simulink model "comparison_amp"  (Simulink 6.0)
settings: Solver=ode45  StartTime=0.0  StopTime=10.0  RelTol=1e-3
undefined symbols (not defined in the file or in its folder): dTypeID, Fs, read, rfdata
libraries: rfports1 x6, simulink x3, rfamplifiers1 x3, rfmathmodels1 x2, dspsnks4 x2, dspmtrx3 x1
settings Model: Creator=ashivapr  LastModifiedBy=rzeng  ProdHWDeviceType=Specified
settings DataIOCC: SaveOutput=off  SaveTime=off  SignalLoggingName=logsOut
settings DebuggingCC: CheckExecutionContextPreStartOutputMsg=on  CheckExecutionContextRuntimeOutputMsg=on  SolverPrmCheckMsg=none
settings HardwareCC: ProdHWDeviceType=Specified
settings ModelReferenceCC: UpdateModelReferenceTargets=IfOutOfDate
settings SFSimCC: SFSimApplyToAllLibs=on  SFSimBuildMode=Incremental

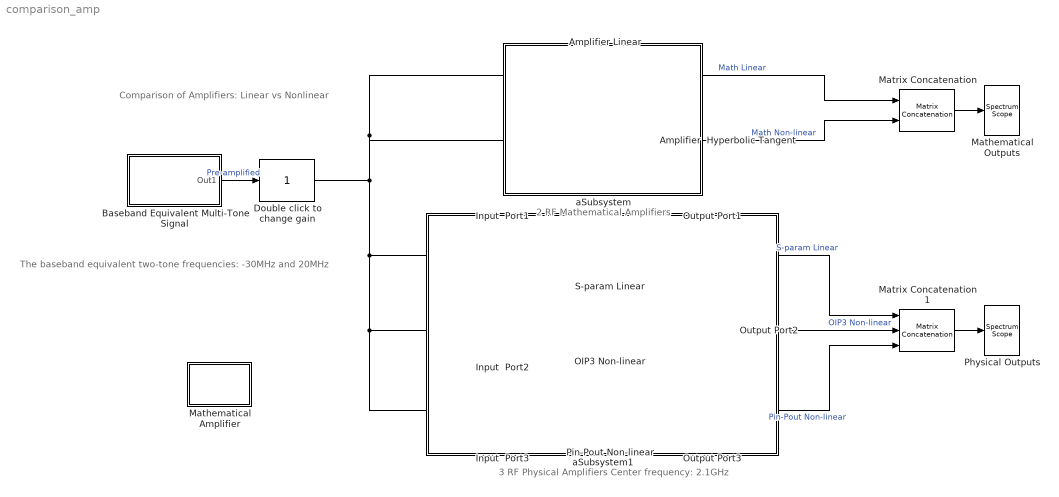
== system comparison_amp ==
  note: Comparison of Amplifiers:
      | Linear vs Nonlinear
  note: 3 RF Physical Amplifiers
      | Center frequency: 2.1GHz
  note: 2 RF Mathematical Amplifiers
  note: The baseband equivalent
      |  two-tone frequencies:
      | -30MHz and 20MHz
  Amplifier  Hyperbolic Tangent : rfmathmodels1/Amplifier  model_select=Hyperbolic tangent  linGaindB=22  GindB=0  iip3=35  am2pm=0  amam=[2.1587 1.1517]  ampm=[4.0033 9.1040]  x=[8.1081 1.5413 6.5202 -0.0718]  y=[4.6645 2.0965 10.88 -0.003]  p=0.5  GoutdB=0  vsat=1  method_select=Noise figure  ntemp=290  nfigure=3.01  nfactor=2  seed=67987
  Amplifier Linear : rfmathmodels1/Amplifier  model_select=Linear  linGaindB=22  GindB=0  iip3=30  am2pm=0  amam=[2.1587 1.1517]  ampm=[4.0033 9.1040]  x=[8.1081 1.5413 6.5202 -0.0718]  y=[4.6645 2.0965 10.88 -0.003]  p=0.5  GoutdB=0  vsat=1  method_select=Noise figure  ntemp=290  nfigure=3.01  nfactor=2  seed=67987
  Baseband Equivalent Multi-Tone Signal : Subsystem  PropExecContextAcrossSSBoundary=on  mask(Baseband Equivalent Multi-Tone Sine Wave){Fc=2.1e9, Frequency=[2.07e9 2.12e9], Amplitude=[0.1 0.05], Phase=[0 pi/4], SampleTime=3e-9, SamplesPerFrame=256}
      mask prompts: Fc "Center frequency (Hz)"; Frequency "Tone frequency (Hz):"; Amplitude "Tone amplitude:"; Phase "Tone phase offset (rad):"; SampleTime "Sample time:"; SamplesPerFrame "Samples per frame:"
      mask help:
      | Generate a baseband equivalent multi-tone complex sinusoid signal. The frequency of the output multi-tone signal is the difference between the Tone frequency and the Center frequency.
      |
      | The values specified here for the Center frequency and Sample time parameters should be equal to the values specified in the 'Input Port' block.
      mask init:
      | if ~isscalar(Fc)
      | 	error('Center frequency must be a scalar');
      | end
      | if ~isnumeric(Frequency)
      | 	error('Tone frequency must be a real vector');
      | end
      | if any(Frequency>=2*Fc)
      | 	error('Tone frequency is too large compared to the Center frequency');
      | end
      | 
      | Frequency = Frequency-Fc;
      mask Display:
      | plot(-0.5,-3,1.5,1,[0:0.005:1], [0.25*sin(2*pi*5*[0:0.005:1])+0.5*sin(2*pi*10*[0:0.005:1]) ]);
      | disp('\nMulti-Tone');
  Double click to change gain : simulink/Math Operations/Slider Gain  low=1  gain=1  high=10
  Input  Port1 : rfports1/Input Port  Description=source block  MaxLength=128  Fc=2.1e9  Ts=3e-9  Zs=50  NoiseFlag=off  seed=67987  GoToTag=BBBCDGBCCQXBBIGOALUIQHV
  Input  Port2 : rfports1/Input Port  Description=source block  MaxLength=128  Fc=2.1e9  Ts=3e-9  Zs=50  NoiseFlag=off  seed=67987  GoToTag=ACCDEHCDDRYCCJHPBMVJRIW
  Input  Port3 : rfports1/Input Port  Description=source block  MaxLength=128  Fc=2.1e9  Ts=3e-9  Zs=50  NoiseFlag=off  seed=67987  GoToTag=BADEFIDEESZDDKIQCNWKSJX
  Mathematical Outputs : dspsnks4/Spectrum Scope  ScopeProperties=on  Domain=Frequency  HorizSpan=1  UseBuffer=off  BufferSize=128  Overlap=64  inpFftLenInherit=off  FFTlength=1024  numAvg=10  DisplayProperties=off  AxisGrid=on  Memory=off  FrameNumber=off  AxisLegend=on  AxisZoom=off  OpenScopeAtSimStart=on  OpenScopeImmediately=off  FigPos=[5 288 496 142]  AxisProperties=off  XUnits=Hertz  XRange=[-Fs/2...Fs/2]  InheritXIncr=on  XIncr=1.0  XLabel=Samples  YUnits=dB  YLabel=Magnitude, dB  LineProperties=off  LineColors=[0 0 0]|[1 0 0]|[0 1 0]
      settings: YMin=-131.600810004824  YMax=51.0081898868428
  Mathematical Amplifier : Subsystem  PropExecContextAcrossSSBoundary=on
      mask Display: disp('Info')
  Matrix Concatenation : simulink/Math Operations/Matrix Concatenation  numInports=2  catMethod=Horizontal
  Matrix Concatenation1 : simulink/Math Operations/Matrix Concatenation  numInports=3  catMethod=Horizontal
  OIP3 Non-linear : rfamplifiers1/General Amplifier  PhysicalDomain=rfsystemsdomain  SubClassName=general-amplifier  LeftPortType=p1  RightPortType=p1  LConnTagsString=__newl0  RConnTagsString=__newr0  RFDATA=read(rfdata.data, 'default.s2p')  InterpMethod=Cubic  IP3Type=OIP3  IIP3=inf  OIP3=30  NF=0  DisplayData=off  PlotFreq=Derived from Input Port parameters  PlotFreqNoSim=Extracted from RFDATA object  Freq=[1.0e9:1.0e8:3e9]  AllPlotType=X-Y plane  NetworkData=S21  PowerData=S11  SmithData=S11  PolarData=S11  ComplexFormat=Magnitude (decibels)  DBFormat=Magnitude (decibels)  PowerFormat=dBm  PhaseFormat=Angle (degrees)  NoneFormat=None
  Output Port1 : rfports1/Output Port  Zl=50  num_Models=1  GoToTag=BBBCDGBCCQXBBIGOALUIQHV  DisplayData=off  PlotFreq=Derived from Input Port parameters  Freq=1e9:1e8:3e9  AllPlotType=Composite data  NoBudgetPlot=Composite data  NetworkData=S11  SmithData=S11  PolarData=S11  ComplexFormat=Magnitude (decibels)  DBFormat=Magnitude (decibels)  DBMFormat=dBm  NoneFormat=None
  Output Port2 : rfports1/Output Port  Zl=50  num_Models=3  GoToTag=ACCDEHCDDRYCCJHPBMVJRIW  DisplayData=off  PlotFreq=Derived from Input Port parameters  Freq=1e9:1e8:3e9  AllPlotType=Composite data  NoBudgetPlot=Composite data  NetworkData=S11  SmithData=S11  PolarData=S11  ComplexFormat=Magnitude (decibels)  DBFormat=Magnitude (decibels)  DBMFormat=dBm  NoneFormat=None
  Output Port3 : rfports1/Output Port  Zl=50  num_Models=3  GoToTag=BADEFIDEESZDDKIQCNWKSJX  DisplayData=off  PlotFreq=Derived from Input Port parameters  Freq=1e9:1e8:3e9  AllPlotType=Composite data  NoBudgetPlot=Composite data  NetworkData=S11  SmithData=S11  PolarData=S11  ComplexFormat=Magnitude (decibels)  DBFormat=Magnitude (decibels)  DBMFormat=dBm  NoneFormat=None
  Physical Outputs : dspsnks4/Spectrum Scope  ScopeProperties=on  Domain=Frequency  HorizSpan=1  UseBuffer=off  BufferSize=128  Overlap=64  inpFftLenInherit=off  FFTlength=1024  numAvg=10  DisplayProperties=off  AxisGrid=on  Memory=off  FrameNumber=off  AxisLegend=on  AxisZoom=off  OpenScopeAtSimStart=on  OpenScopeImmediately=off  FigPos=[508 287 501 144]  AxisProperties=off  XUnits=Hertz  XRange=[-Fs/2...Fs/2]  InheritXIncr=on  XIncr=1.0  XLabel=Samples  YUnits=dB  YLabel=Magnitude, dB  LineProperties=off  LineColors=[0 0 0]|[1 0 0]|[0 1 0]
      settings: YMin=-131.600810004824  YMax=51.0081898868428
  Pin-Pout Non-linear : rfamplifiers1/General Amplifier  PhysicalDomain=rfsystemsdomain  SubClassName=general-amplifier  LeftPortType=p1  RightPortType=p1  LConnTagsString=__newl0  RConnTagsString=__newr0  RFDATA=read(rfdata.data, 'default.amp')  InterpMethod=Cubic  IP3Type=OIP3  IIP3=inf  OIP3=30  NF=0  DisplayData=off  PlotFreq=Derived from Input Port parameters  PlotFreqNoSim=Extracted from RFDATA object  Freq=[1.0e9:1.0e8:3e9]  AllPlotType=X-Y plane  NetworkData=S21  PowerData=S11  SmithData=S11  PolarData=S11  ComplexFormat=Magnitude (decibels)  DBFormat=Magnitude (decibels)  PowerFormat=dBm  PhaseFormat=Angle (degrees)  NoneFormat=None
  S-param Linear : rfamplifiers1/General Amplifier  PhysicalDomain=rfsystemsdomain  SubClassName=general-amplifier  LeftPortType=p1  RightPortType=p1  LConnTagsString=__newl0  RConnTagsString=__newr0  RFDATA=read(rfdata.data, 'default.s2p')  InterpMethod=Cubic  IP3Type=OIP3  IIP3=inf  OIP3=inf  NF=0  DisplayData=off  PlotFreq=Derived from Input Port parameters  PlotFreqNoSim=Extracted from RFDATA object  Freq=[1.0e9:1.0e8:3e9]  AllPlotType=X-Y plane  NetworkData=S21  PowerData=S11  SmithData=S11  PolarData=S11  ComplexFormat=Magnitude (decibels)  DBFormat=Magnitude (decibels)  PowerFormat=dBm  PhaseFormat=Angle (degrees)  NoneFormat=None
  aSubsystem : Subsystem  PropExecContextAcrossSSBoundary=on
      mask Display: disp('')
  aSubsystem1 : Subsystem  PropExecContextAcrossSSBoundary=on
      mask Display: disp('')
  wires:
  Baseband Equivalent Multi-Tone Signal/1(Out1) -> Double click to change gain/1  "Pre-amplified"
  Amplifier  Hyperbolic Tangent/1 -> Matrix Concatenation/2  "Math Non-linear"
  Matrix Concatenation/1 -> Mathematical Outputs/1
  Output Port1/1 -> Matrix Concatenation1/1  "S-param Linear"
  Amplifier Linear/1 -> Matrix Concatenation/1  "Math Linear"
  Matrix Concatenation1/1 -> Physical Outputs/1
  Output Port3/1 -> Matrix Concatenation1/3  "Pin-Pout Non-linear"
  Output Port2/1 -> Matrix Concatenation1/2  "OIP3 Non-linear"
  Double click to change gain/1 -> Amplifier Linear/1, Amplifier  Hyperbolic Tangent/1, Input  Port1/1, Input  Port3/1, Input  Port2/1
  connections:
  Input  Port1/RConn1 -- S-param Linear/LConn1
  S-param Linear/RConn1 -- Output Port1/LConn1
  Input  Port2/RConn1 -- OIP3 Non-linear/LConn1
  Input  Port3/RConn1 -- Pin-Pout Non-linear/LConn1
  Pin-Pout Non-linear/RConn1 -- Output Port3/LConn1
  OIP3 Non-linear/RConn1 -- Output Port2/LConn1

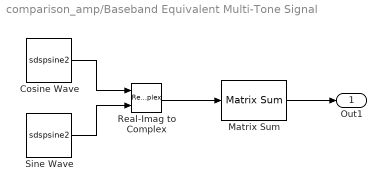
== system comparison_amp/Baseband Equivalent Multi-Tone Signal ==
  Cosine Wave : S-Function  AncestorBlock=dspsrcs4/Sine Wave  FunctionName=sdspsine2  Parameters=Amplitude,Frequency,Phase,SampleMode,OutComplex,CompMethod,SampleTime,SamplesPerFrame,ResetState,TableSize,isCustomFloat,isSigned,dTypeID,wordLength,fracBits  mask(Sine Wave){Amplitude=Amplitude, Frequency=Frequency, Phase=Phase+(pi/2), SampleMode=Discrete, OutComplex=Real, CompMethod=Trigonometric fcn, TableSize=Speed, SampleTime=SampleTime, SamplesPerFrame=SamplesPerFrame, additionalParams=off, allowOverrides=on, dataType=double, wordLen=16, udDataType=sfix(16), fracBitsMode=Best precision, numFracBits=15, ResetState=Restart at time zero}
      mask prompts: Frequency "Frequency (Hz):"; Phase "Phase offset (rad):"; SampleMode "Sample mode:"; OutComplex "Output complexity:"; CompMethod "Computation method:"; TableSize "Optimize table for:"; SampleTime "Sample time:"; SamplesPerFrame "Samples per frame:"; additionalParams "------- Show additional parameters --------"; allowOverrides "Allow overrides from DSP Fixed-Point Attributes blocks"; dataType "Output data type:"; wordLen "Word length:"; udDataType "User-defined data type (e.g. sfix(16), float('single')):"; fracBitsMode "Set fraction length in output to:"; numFracBits "Fraction length:"; ResetState "State when re-enabled:"
      mask help: Output samples of a sinusoid. To generate more than one sinusoid simultaneously, enter a vector of values for the amplitude, frequency, and phase parameters.
      mask init:
      | [x,y] = dspblksine('icon');
      | [dtInfo,dTypeID]=dspblksine('init');
      | isSigned=dtInfo.DataTypeIsSigned;
      | isCustomFloat=dtInfo.DataTypeIsCustomFloat;
      | wordLength=dtInfo.DataTypeWordLength;
      | fracBits=dtInfo.DataTypeFracOrMantBits;
      | dType=dataType;
      mask Help: web(dspbhelp);
      mask StyleString: edit,edit,edit,popup(Discrete|Continuous),popup(Real|Complex),popup(Trigonometric fcn|Table lookup|Differential),popup(Speed|Memory),edit,edit,checkbox,checkbox,popup(double|single|Fixed-point|User-defined|Inherit via back propagation),edit,edit,popup(Best precision|User-defined),edit,popup(Restart at time zero|Catch up to simulation time)
      mask CallbackString: |||dspblksine;||dspblksine;||||dspblksine|dspblksine|dspblksine||dspblksine|dspblksine||
      mask Display:
      | plot(x,y)
      | text(3.25,.75,'DSP');
  Matrix Sum : dspmtrx3/Matrix Sum  DialogController=dspDDGCreate  DialogControllerArgs=DataTag0  Dim=Rows  roundingMode=Floor  overflowMode=off
  Real-Imag to Complex : RealImagToComplex
  Sine Wave : S-Function  AncestorBlock=dspsrcs4/Sine Wave  FunctionName=sdspsine2  Parameters=Amplitude,Frequency,Phase,SampleMode,OutComplex,CompMethod,SampleTime,SamplesPerFrame,ResetState,TableSize,isCustomFloat,isSigned,dTypeID,wordLength,fracBits  mask(Sine Wave){Amplitude=Amplitude, Frequency=Frequency, Phase=Phase, SampleMode=Discrete, OutComplex=Real, CompMethod=Trigonometric fcn, TableSize=Speed, SampleTime=SampleTime, SamplesPerFrame=SamplesPerFrame, additionalParams=off, allowOverrides=on, dataType=double, wordLen=16, udDataType=sfix(16), fracBitsMode=Best precision, numFracBits=15, ResetState=Restart at time zero}
      mask prompts: Frequency "Frequency (Hz):"; Phase "Phase offset (rad):"; SampleMode "Sample mode:"; OutComplex "Output complexity:"; CompMethod "Computation method:"; TableSize "Optimize table for:"; SampleTime "Sample time:"; SamplesPerFrame "Samples per frame:"; additionalParams "------- Show additional parameters --------"; allowOverrides "Allow overrides from DSP Fixed-Point Attributes blocks"; dataType "Output data type:"; wordLen "Word length:"; udDataType "User-defined data type (e.g. sfix(16), float('single')):"; fracBitsMode "Set fraction length in output to:"; numFracBits "Fraction length:"; ResetState "State when re-enabled:"
      mask help: Output samples of a sinusoid. To generate more than one sinusoid simultaneously, enter a vector of values for the amplitude, frequency, and phase parameters.
      mask init: same as comparison_amp/Baseband Equivalent Multi-Tone Signal/Cosine Wave
      mask Help: web(dspbhelp);
      mask StyleString: edit,edit,edit,popup(Discrete|Continuous),popup(Real|Complex),popup(Trigonometric fcn|Table lookup|Differential),popup(Speed|Memory),edit,edit,checkbox,checkbox,popup(double|single|Fixed-point|User-defined|Inherit via back propagation),edit,edit,popup(Best precision|User-defined),edit,popup(Restart at time zero|Catch up to simulation time)
      mask CallbackString: |||dspblksine;||dspblksine;||||dspblksine|dspblksine|dspblksine||dspblksine|dspblksine||
      mask Display:
      | plot(x,y)
      | text(3.25,.75,'DSP');
  Out1 : Outport
  wires:
  Real-Imag to Complex/1 -> Matrix Sum/1
  Sine Wave/1 -> Real-Imag to Complex/2
  Cosine Wave/1 -> Real-Imag to Complex/1
  Matrix Sum/1 -> Out1/1

== system comparison_amp/Mathematical Amplifier ==
  note: Comparison of Amplifiers: Linear vs Nonlinear
      |
      | The RF Blockset has two kinds of amplifier blocks: mathematical and physical amplifiers.
      |
      | This demo shows the two-tone intermodulation performance of
      | 2 mathematical amplifiers and 3 physical amplifiers:
      |
      | Math Linear: described by a linear gain and noise figure
      |
      | Math Non-linear: tanh model using input-referenced IP3
      |
      | S-para Linear: described by the S-parameters in 'default.s2p' file
      |
      | OIP3 Non-linear: described by the S-parameters in 'default.s2p' file and OIP3 parameter
      |
      | Pin-Pout Non-linear: described by the S-parameters and Pin-Pout date in 'default.amp' file
      |
      | To view the intermodulation performance at the outputs,
      | double click the 'Slider Gain' block and change the value of the gain
      | while the model is running.

== system comparison_amp/aSubsystem ==

== system comparison_amp/aSubsystem1 ==
